simulink model "untitled"  (Simulink 7.7)
settings: Solver=FixedStepDiscrete  StartTime=0.0  StopTime=.524288  FixedStep=2e-6  RelTol=1e-3
undefined symbols (not defined in the file or in its folder): dfilt, fdesignblkfcn, gcbh, get, One, sided
libraries: simulink_extras x2, dspsnks4 x2, commnoisgen2 x1, dsparch4 x1
settings Model: Creator=ArunKB  LastModifiedBy=ArunKB  SimulationMode=accelerator

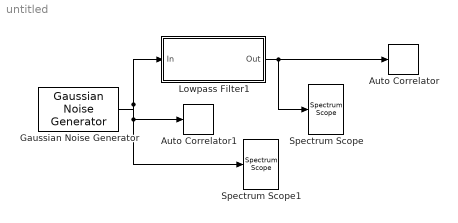
== system untitled ==
  Auto Correlator : simulink_extras/Additional Sinks/Auto Correlator  SystemSampleTime=-1  npts=100  HowOften=50  sampleT=2e-6
  Auto Correlator1 : simulink_extras/Additional Sinks/Auto Correlator  SystemSampleTime=-1  npts=100  HowOften=50  sampleT=2e-6
  Gaussian Noise Generator : commnoisgen2/Gaussian Noise Generator  SystemSampleTime=-1  m=0  d=1  s=41  Ts=2e-6  frameBased=off  sampPerFrame=1  orient=off  outDataType=double
  Lowpass Filter1 : Subsystem  DialogController=fdesignblkfcn  DialogControllerArgs=DataTag1  InitFcn=fdesignblkfcn(gcbh, {'InitFcn'});
      settings: CopyFcn=fdesignblkfcn(gcbh, {'CopyFcn'});
      mask Type: Lowpass Filter
      mask Description: Design a lowpass filter
      mask Help: helpview(mapfilelocation('dsp'), 'dsplowpassfilter');
      mask Display: disp('Lowpass')
  Spectrum Scope : dspsnks4/Spectrum Scope  SystemSampleTime=-1  ScopeProperties=on  Domain=Frequency  HorizSpan=1  UseBuffer=on  BufferSize=262144  Overlap=0  TreatMby1Signals=One channel  inpFftLenInherit=on  FFTlength=262144  numAvg=1  DisplayProperties=off  AxisGrid=on  Memory=off  FrameNumber=on  AxisLegend=off  AxisZoom=off  OpenScopeAtSimStart=on  OpenScopeImmediately=off  FigPos=get(0,'defaultfigureposition')  AxisProperties=off  XUnits=Hertz  XRange=One-sided ([0...Fs/2])  XDisplay=0  InheritXIncr=on  XIncr=1.0  XLabel=Samples  XLimit=Auto  YUnits=dBW/Hertz  XMax=1  XMin=0  YLabel=Magnitude-squared, dB  LineProperties=off  wintypeSpecScope=Boxcar  RsSpecScope=50  betaSpecScope=5  winsampSpecScope=Periodic  XAxisParamsVer=6.9  isFrameUpgraded=on
      settings: YMin=-10  YMax=10
  Spectrum Scope1 : dspsnks4/Spectrum Scope  SystemSampleTime=-1  ScopeProperties=on  Domain=Frequency  HorizSpan=1  UseBuffer=on  BufferSize=262144  Overlap=0  TreatMby1Signals=One channel  inpFftLenInherit=on  FFTlength=262144  numAvg=1  DisplayProperties=off  AxisGrid=on  Memory=off  FrameNumber=on  AxisLegend=off  AxisZoom=off  OpenScopeAtSimStart=on  OpenScopeImmediately=off  FigPos=get(0,'defaultfigureposition')  AxisProperties=off  XUnits=Hertz  XRange=One-sided ([0...Fs/2])  XDisplay=0  InheritXIncr=on  XIncr=1.0  XLabel=Samples  XLimit=Auto  YUnits=dBW/Hertz  XMax=1  XMin=0  YLabel=Magnitude-squared, dB  LineProperties=off  wintypeSpecScope=Boxcar  RsSpecScope=50  betaSpecScope=5  winsampSpecScope=Periodic  XAxisParamsVer=6.9  isFrameUpgraded=on
      settings: YMin=-10  YMax=10
  wires:
  Gaussian Noise Generator/1 -> Lowpass Filter1/1(In), Spectrum Scope1/1, Auto Correlator1/1
  Lowpass Filter1/1(Out) -> Spectrum Scope/1, Auto Correlator/1

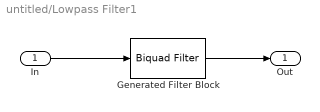
== system untitled/Lowpass Filter1 ==
  In : Inport
  Generated Filter Block : dsparch4/Biquad Filter  Tag=BlockMethodSubSystem  IIRFiltStruct=Direct form I transposed  CoeffSource=Specify via dialog  BiQuadCoeffs=[0.352301465508541 0.704602931017083 0.352301465508541 1 -0.180628612762935 0.530389262111784;0.372445789009338 0.744891578018675 0.372445789009338 1 -0.136933364406744 0.160178043264713;0.298552689881353 0.597105379762706 0.298552689881353 1 -0.120325317460228 0.0194651389091043;0.471597057189982 0.471597057189982 0 1 -0.0592209128889308 0;0.287579135141555 0.575158270283109 0.287579135141555 1 -0.126220781831806 0.0694148962117701;0.127150102249276 0.254300204498551 0.127150102249276 1 -0.154075206809667 0.305413569048635;0.257691807936424 0.515383615872848 0.257691807936424 1 -0.222201170929932 0.882615831557847;0.383717151997119 0.767434303994237 0.383717151997119 1 -0.165908942393244 0.405675767770967;0.424194504367503 0.848389008735007 0.424194504367503 1 -0.13089759638918 0.109039552959184;0.300731101429764 0.601462202859527 0.300731101429764 1 -0.118908998066904 0.00746526824571344;0.270051771137896 0.540103542275793 0.270051771137896 1 -0.122736195391717 0.0398914802410605;0.223834597757338 0.447669195514675 0.223834597757338 1 -0.144556227263978 0.224763311815564;0.415266362341515 0.830532724683031 0.415266362341515 1 -0.199023214159024 0.68623888098888]  a0Flag=Warning  IC=0  ICnum=0  ICden=0  InputProcessing=Columns as channels (frame based)  denAccumFracLength=30  denProdOutputFracLength=30  secondMemoryFracLength=15  roundingMode=Floor  overflowMode=off  ScaleValues=[0.465985780077502;1;1;1;1;1;1;1;1;1;1;1;1;1]  optimizeScaleValues=off  ScaleValueMode=Specify via input port (g)  scaleValueFracLength=14  FilterSource=Specify via dialog  dfiltObjectName=dfilt.df2tsos([1 0.3 0.4],[1 0.1 0.2])
  Out : Outport
  wires:
  Generated Filter Block/1 -> Out/1
  In/1 -> Generated Filter Block/1
